simulink library "ammclib_bam_S32K3xx"  (R2016a)
settings: Solver=VariableStepAuto  SolverMode=SingleTasking  StartTime=0.0  StopTime=10.0  RelTol=1e-3
(part 1 of 50)
settings Model: Creator=B37097  LastModifiedBy=B37097
settings DataIOCC: ReturnWorkspaceOutputs=on
settings DebuggingCC: SFUnexpectedBacktrackingDiag=error  SFNoUnconditionalDefaultTransitionDiag=error
settings SFSimCC: SimUseLocalCustomCode=on
settings RTWCC: RTWUseLocalCustomCode=on
settings GRTTargetCC: TargetLangStandard=C99 (ISO)  GeneratePreprocessorConditionals=Use local settings
settings ConfigComp: CovMetricSettings=dwe  CovHtmlReporting=off  CovSaveCumulativeToWorkspaceVar=off  CovSaveSingleToWorkspaceVar=off  CovExternalEMLEnable=on

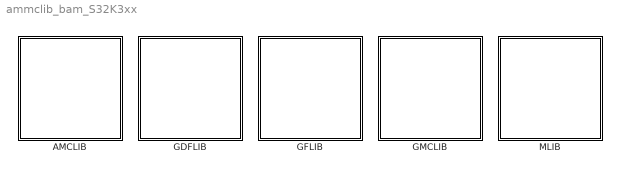
== system ammclib_bam_S32K3xx ==
  AMCLIB : Subsystem
  GDFLIB : Subsystem
  GFLIB : Subsystem
  GMCLIB : Subsystem
  MLIB : Subsystem

== system ammclib_bam_S32K3xx/AMCLIB ==
  F16 : Subsystem
  F32 : Subsystem
  FLT : Subsystem

== system ammclib_bam_S32K3xx/GDFLIB ==
  F16 : Subsystem
  F32 : Subsystem
  FLT : Subsystem

== system ammclib_bam_S32K3xx/GFLIB ==
  F16 : Subsystem
  F32 : Subsystem
  FLT : Subsystem

== system ammclib_bam_S32K3xx/GMCLIB ==
  F16 : Subsystem
  F32 : Subsystem
  FLT : Subsystem
  Generic : Subsystem

== system ammclib_bam_S32K3xx/MLIB ==
  F16 : Subsystem
  F32 : Subsystem
  F32F16F16 : Subsystem
  FLT : Subsystem
